simulink model "activeSuspensionModel"  (R2016a)
settings: Solver=VariableStepAuto  StartTime=0.0  StopTime=15.0  RelTol=1e-3
values from neighbouring files (symbols this model uses):
  Ad = [1 T 0 -T ... (first row only)    [linearRegression.m]
  Bd = [0 0 ... (first row only)    [linearRegression.m]
  Cd = [1 0 0 0 ... (first row only)    [linearRegression.m]
  Dd = [0 0 ... (first row only)    [linearRegression.m]
  T = 0.002    [linearRegression.m]    (also in simPlantMPC.m)
undefined symbols (not defined in the file or in its folder): K
settings Model: Creator=JMH  LastModifiedBy=JMH
settings GRTTargetCC: GeneratePreprocessorConditionals=Use local settings

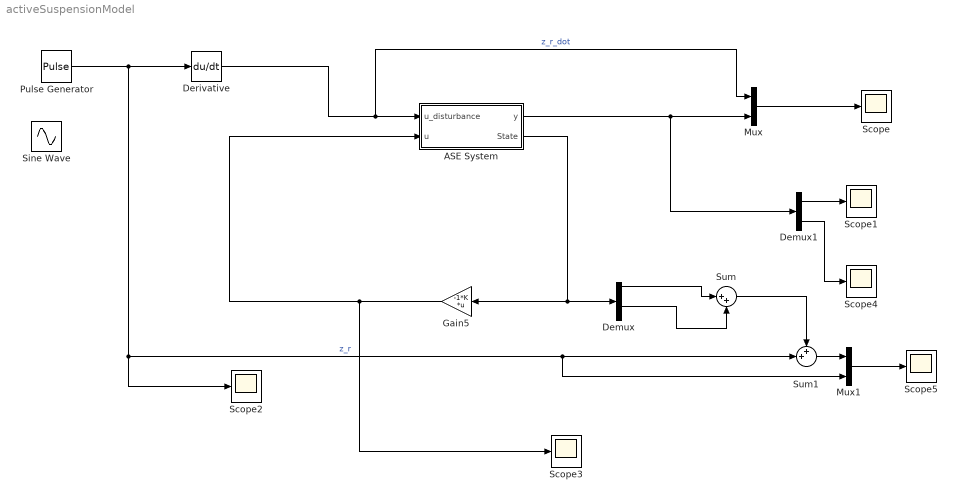
== system activeSuspensionModel ==
  ASE System : Subsystem
  Demux : Demux
  Demux1 : Demux  Outputs=2
  Derivative : Derivative
  Gain5 : Gain  Gain=-1*K  Multiplication=Matrix(K*u)
  Mux : Mux  Inputs=2
  Mux1 : Mux  Inputs=2
  Pulse Generator : DiscretePulseGenerator  PulseType=Time based  Amplitude=0.01  Period=10/3  PulseWidth=20
  Scope{,1..5} (6 alike) : Scope
  Sine Wave : Sin  Amplitude=0.01  Frequency=3*pi/5  SampleTime=0
  Sum : Sum  Inputs=|++
  Sum1 : Sum  Inputs=++|
  wires:
  Gain5/1 -> Scope3/1, ASE System/2(u)
  Derivative/1 -> Mux/1, ASE System/1(u_disturbance)  "z_r_dot"
  ASE System/2(State) -> Demux/1, Gain5/1
  ASE System/1(y) -> Demux1/1, Mux/2
  Mux/1 -> Scope/1
  Demux1/1 -> Scope1/1
  Demux1/2 -> Scope4/1
  Pulse Generator/1 -> Mux1/2, Sum1/2, Scope2/1, Derivative/1  "z_r"
  Demux/1 -> Sum/1
  Demux/3 -> Sum/2
  Sum/1 -> Sum1/1
  Sum1/1 -> Mux1/1
  Mux1/1 -> Scope5/1

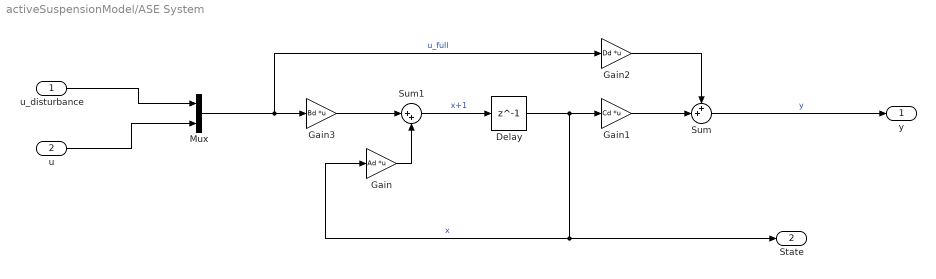
== system activeSuspensionModel/ASE System ==
  u_disturbance : Inport
  u : Inport  Port=2
  Delay : Delay  DelayLength=1  SampleTime=T
  Gain : Gain  Gain=Ad  Multiplication=Matrix(K*u)
  Gain1 : Gain  Gain=Cd  Multiplication=Matrix(K*u)
  Gain2 : Gain  Gain=Dd  Multiplication=Matrix(K*u)
  Gain3 : Gain  Gain=Bd  Multiplication=Matrix(K*u)
  Mux : Mux  Inputs=2
  Sum : Sum  Inputs=++|
  Sum1 : Sum  Inputs=|++
  y : Outport
  State : Outport  Port=2
  wires:
  Gain2/1 -> Sum/1
  Gain1/1 -> Sum/2
  Sum/1 -> y/1  "y"
  Gain/1 -> Sum1/2
  u/1 -> Mux/2
  u_disturbance/1 -> Mux/1
  Gain3/1 -> Sum1/1
  Mux/1 -> Gain2/1, Gain3/1  "u_full"
  Delay/1 -> State/1, Gain/1, Gain1/1  "x"
  Sum1/1 -> Delay/1  "x+1"
